simulink model "mean_wind_fluctuations"  (R2018a)
settings: Solver=VariableStepAuto  StartTime=0.0  StopTime=1000  RelTol=1e-3
values from neighbouring files (symbols this model uses):
  my = 0.001    [wind.m]
libraries: simulink x1
settings Model: Creator=revolt  LastModifiedBy=revolt

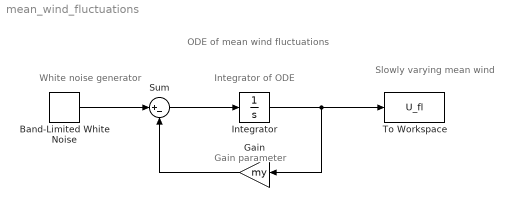
== system mean_wind_fluctuations ==
  note: ODE of mean wind fluctuations
  note: Integrator of ODE
  note: Slowly varying mean wind
  note: White noise generator
  note: Gain parameter
  Band-Limited White Noise : simulink/Sources/Band-Limited White Noise  Cov=w  Ts=1  seed=[23341]
  Gain : Gain  Gain=my
  Integrator : Integrator
  Sum : Sum  Inputs=|+-
  To Workspace : ToWorkspace  VariableName=U_fl  SaveFormat=Timeseries  SampleTime=-1
  wires:
  Band-Limited White Noise/1 -> Sum/1
  Sum/1 -> Integrator/1
  Integrator/1 -> Gain/1, To Workspace/1
  Gain/1 -> Sum/2
